simulink model "Quiz4_PartD_SimBlock"  (R2017b)
settings: Solver=FixedStepAuto  StartTime=0.0  StopTime=30  FixedStep=.05  RelTol=1e-3
model workspace (MAT data in the model file):
  Z = 0.01
  b = 2000
  k = 50000
  m = 3000
  phi = 1.57079632679
  w = 3
settings Model: Creator=Harrison  LastModifiedBy=Harrison
settings DataIOCC: SaveFormat=Array

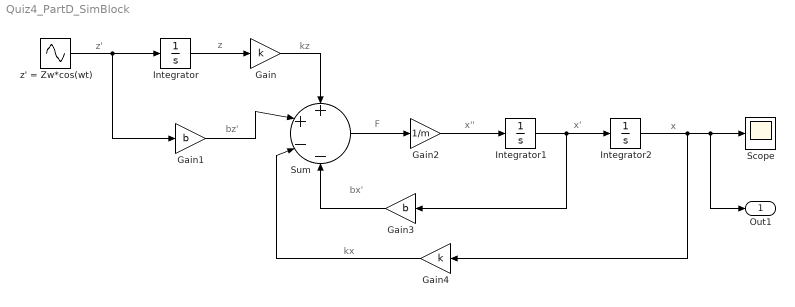
== system Quiz4_PartD_SimBlock ==
  note: F
  note: kz
  note: bz'
  note: kx
  note: bx'
  note: x
  note: x'
  note: x''
  note: z
  note: z'
  Gain : Gain  Gain=k
  Gain1 : Gain  Gain=b
  Gain2 : Gain  Gain=1/m
  Gain3 : Gain  Tag=b  Gain=b
  Gain4 : Gain  Gain=k
  Integrator : Integrator
  Integrator1 : Integrator
  Integrator2 : Integrator
  Scope : Scope
  Sum : Sum  Inputs=++--
  z' = Zw*cos(wt) : Sin  Amplitude=Z*w  Frequency=w  Phase=phi  SampleTime=0
  Out1 : Outport
  wires:
  z' = Zw*cos(wt)/1 -> Gain1/1, Integrator/1
  Integrator/1 -> Gain/1
  Gain/1 -> Sum/1
  Gain1/1 -> Sum/2
  Sum/1 -> Gain2/1
  Integrator1/1 -> Gain3/1, Integrator2/1
  Gain2/1 -> Integrator1/1
  Gain3/1 -> Sum/4
  Integrator2/1 -> Gain4/1, Out1/1, Scope/1
  Gain4/1 -> Sum/3
